simulink model "DT_enviroment_state_machine_llm_udp_simscape"  (R2026a)
settings: Solver=ode23t  StopTime=120.500  FixedStep=1e-3
InitFcn:
  | V_bias_cmd=0;
  | enable_cmd=0;
  | mode_cmd=0;
  | P_batt_cmd=0;
libraries: fl_lib x14, nesl_utility x12, batteryecm_lib x2, eeGeneralControl x2, slpidlib x2
(part 1 of 2)
settings Model: Creator=Peska  LastModifiedBy=thienan
settings DebuggingCC: SaveWithParameterizedLinksMsg=none
settings SimscapeCC: SimscapeLogType=none  SimscapeLogDataHistory=5000.0

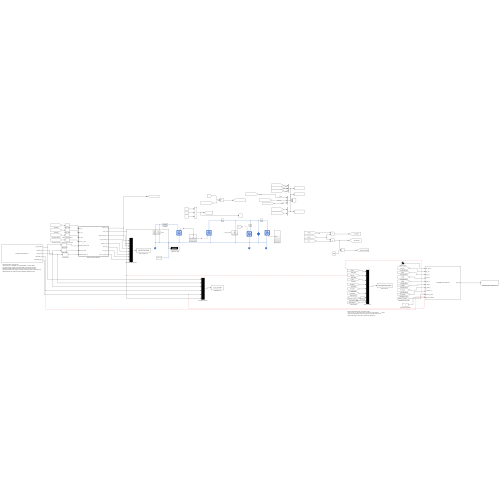
[thumbnail: Simulink's stored preview of the top-level diagram]
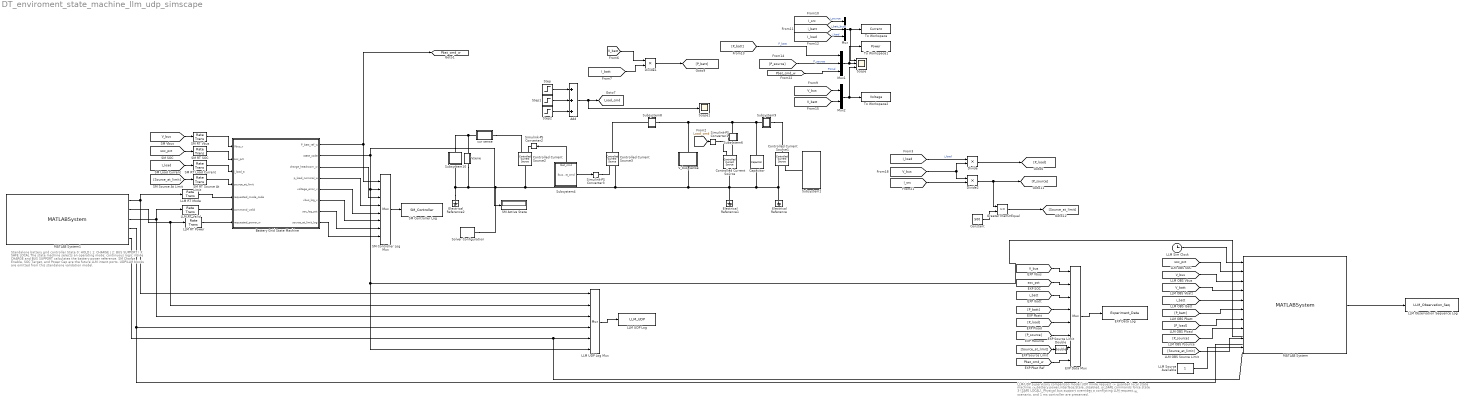
== system DT_enviroment_state_machine_llm_udp_simscape ==
  note: Standalone battery grid controller
      | State 0: HOLD | 1: CHARGE | 2: BUS SUPPORT | 3: SAFE LOCAL
      | The state machine selects an operating mode; continuous logic inside
      | CHARGE and BUS SUPPORT calculates the battery power reference.
      | SM Charge Enable, SOC Target, and Power Cap are the future LLM intent ports.
      | UDP/LLM blocks are omitted from this standalone validation model.
  note: Instrumented deterministic comparison model
      | This is a copy; DT_enviroment_state_machine.slx is unchanged.
      | The plant, state machine, scenario, and 1 ms controller are preserved.
  note: LLM/UDP supervisory comparison model
      | UDP mode request -> guarded local state machine -> battery power interface
      | Stale, disabled, or SAFE commands force state 3 (SAFE LOCAL).
      | Physical bus support overrides a conflicting LLM request.
  Add : Sum  Inputs=+++
  Battery Grid State Machine : MATLAB Function  TreatAsAtomicUnit=on
  Capacitor : fl_lib/Electrical/Electrical Elements/Capacitor  c=5e-3 F  r=1e-6 Ohm  g=0 1/Ohm  i_specify=off  i_priority=None  i=0 A  i_nominal_specify=off  i_nominal_value=1  i_nominal_unit=A  v_specify=off  v_priority=High  v=400 V  v_nominal_specify=off  v_nominal_value=1  v_nominal_unit=V  vc_specify=on  vc_priority=High  vc=400 V  vc_nominal_specify=off  vc_nominal_value=400  vc_nominal_unit=V
  Constant : Constant  Value=500
  Controlled Current Source{,1..3} (4 alike) : fl_lib/Electrical/Electrical Sources/Controlled Current Source
  Divide : Product  Inputs=**
  Divide1 : Product  Inputs=**
  Divide2 : Product  Inputs=**
  EXP Data Log : ToWorkspace  VariableName=Experiment_Data  SaveFormat=Structure With Time  SampleTime=-1
  EXP Data Mux : Mux  Inputs=8
  EXP Source Limit Double : DataTypeConversion  OutDataTypeStr=double  SaturateOnIntegerOverflow=off  RndMeth=Floor
  Electrical Reference : fl_lib/Electrical/Electrical Elements/Electrical Reference
  Electrical Reference1 : fl_lib/Electrical/Electrical Elements/Electrical Reference
  Electrical Reference2 : fl_lib/Electrical/Electrical Elements/Electrical Reference
  GreaterThanOrEqual : RelationalOperator  OutDataTypeStr=boolean  RndMeth=Simplest  InputSameDT=off
  LLM Observation Sequence Log : ToWorkspace  VariableName=LLM_Observation_Seq  SaveFormat=Structure With Time  SampleTime=-1
  LLM RT Mode : RateTransition  OutPortSampleTime=1e-3
  LLM RT Power : RateTransition  OutPortSampleTime=1e-3
  LLM RT Valid : RateTransition  OutPortSampleTime=1e-3
  LLM Sim Clock : Clock
  LLM Source Available : Constant
  LLM UDP Log : ToWorkspace  VariableName=LLM_UDP  SaveFormat=Structure With Time  SampleTime=-1
  LLM UDP Log Mux : Mux  Inputs=6
  MATLAB System : MATLABSystem  System=DTUdpObservationSender  RemoteHost=127.0.0.1  RemotePort=55001  SourceName=simulink  SampleDecimation=1  SourcePowerLimitW=NaN  MaxSafeChargeW=NaN
      mask Type: DTUdpObservationSender
  MATLAB System1 : MATLABSystem  System=DTUdpCommandReceiver  LocalPort=55000  DefaultPCommandW=0  DefaultEnable=on  DefaultModeCode=0  MaxCommandAgeS=10
      mask Type: DTUdpCommandReceiver
  Mux : Mux  Inputs=3
  Mux1 : Mux  Inputs=3
  Mux2 : Mux  Inputs=2
  SM Active State : Display
  SM Controller Log : ToWorkspace  VariableName=SM_Controller  SaveFormat=Structure With Time  SampleTime=-1
  SM Controller Log Mux : Mux  Inputs=8
  SM RT Load Current : RateTransition  OutPortSampleTime=1e-3
  SM RT SOC : RateTransition  OutPortSampleTime=1e-3
  SM RT Source At Limit : RateTransition  OutPortSampleTime=1e-3
  SM RT Vbus : RateTransition  OutPortSampleTime=1e-3
  Scope : Scope  NumInputPorts=3
      settings: TimeSpan=200  ActiveDisplayYMinimum=-1.87953  ActiveDisplayYMaximum=1.91579
  Scope1 : Scope
      settings: ActiveDisplayYMinimum=0.40625  ActiveDisplayYMaximum=1.34375
  Simulink-PS Converter1 : nesl_utility/Simulink-PS Converter  PhysicalDomain=network_engine_domain  SubClassName=ps_input  LeftPortType=input  RightPortType=output  PseudoPeriodic=off  Frequencies=[]  NoiseDistribution=none  NoiseParameters=[]  Unit=1  AffineConversion=off  FilteringAndDerivatives=provide  SimscapeFilterOrder=1  InputFilterTimeConstant=0.001  UdotUserProvided=0
  Simulink-PS Converter2 : nesl_utility/Simulink-PS Converter  PhysicalDomain=network_engine_domain  SubClassName=ps_input  LeftPortType=input  RightPortType=output  PseudoPeriodic=off  Frequencies=[]  NoiseDistribution=none  NoiseParameters=[]  Unit=1  AffineConversion=off  FilteringAndDerivatives=provide  SimscapeFilterOrder=1  InputFilterTimeConstant=0.001  UdotUserProvided=0
  Simulink-PS Converter3 : nesl_utility/Simulink-PS Converter  PhysicalDomain=network_engine_domain  SubClassName=ps_input  LeftPortType=input  RightPortType=output  PseudoPeriodic=off  Frequencies=[]  NoiseDistribution=none  NoiseParameters=[]  Unit=1  AffineConversion=off  FilteringAndDerivatives=provide  SimscapeFilterOrder=1  InputFilterTimeConstant=0.001  UdotUserProvided=0
  Solver Configuration : nesl_utility/Solver Configuration  PhysicalDomain=network_engine_domain  SubClassName=solver  LeftPortType=input  RightPortType=generic  Tones=[]  Harmonics=[]  SimulateNoise=off  Profile=off  UseLocalSampling=off  EnableSwitchedLinearOptims=on  FrequencyDomain=off  UseCCode=off  RelTol=0.001  AbsTol=0.001  MinStep=1e-09  ToWorkspace=off  RevertToSquareIcSolve=off  NumHomotopyIterations=100  PhasorMode=off  PhasorModeNumHarmonics=1  ConsistencySolver=NEWTON_XTOL_AFTER_FTOL  CanonicalOrdering=UNORDERED  OptimizeIntermediates=UNOPTIMIZED  IndexReductionMethod=DerivativeReplacement  DoDC=off  ResidualTolerance=1e-09  ConsistencyTolSource=GLOBAL  ConsistencyAbsTol=0.001  ConsistencyRelTol=0.001  ConsistencyTolFactor=0.001  UseLocalSolver=off  LocalSolverChoice=NE_BACKWARD_EULER_ADVANCER  ResolveIndetEquations=on  FunctionEvalNumThread=1  LocalSolverSampleTime=0.001  DoFixedCost=off  MaxNonlinIter=3  MaxModeIter=2  ComputeImpulses=off  ImpulseIterations=2  LinearAlgebra=auto  LinearAlgebraNumThread=0  EquationFormulation=NE_TIME_EF  DelaysMemoryBudget=1024  AutomaticFiltering=on  FilteringTimeConstant=0.001  PartitionStorageMethod=AS_NEEDED  PartitionMemoryBudget=1024  PartitionMethod=ROBUST  MultibodyUseLocalSolver=off  MultibodyLocalSolverChoice=ODE1  MultibodyLocalSolverSampleTime=0.001
  Step : Step  Time=50  InitialValue=0.5  FinalValue=1.25  SampleTime=0
  Step1 : Step  Time=100  FinalValue=0.25  SampleTime=0
  Step2 : Step  Time=160  FinalValue=-1  SampleTime=0
  Subsystem1 : Subsystem
  Subsystem10 : Subsystem
  Subsystem4 : Subsystem
      settings: PortSchema="{\"entries\":[{\"content\":{\"sides\":[{\"content\":{},\"type\":\"ConnectorPlacement.EquallySpacedRectSide\",\"uuid\":\"6a1a1ce4-53ed-4982-894a-a22a93ba5ab9\"},{\"content\":{\"connectorIds\":[\"Out1\"],\"side\":\"RIGHT\"},\"type\":\"ConnectorPlacement.EquallySpacedRectSide\",\"uuid\":\"d093341d-d8fd-41c9-a305-3247a499ae5f\"},{\"content\":{\"connectorIds\":[\"Out2\"],\"side\":\"TOP\"},\"type\":\"ConnectorPlacement.EquallySpacedRectSide\",\"uuid\":\"086192a8-14eb-4f6e-a910-e0970e09cefc\"}]},\"type\":\"ConnectorPlacement.EquallySpacedConnector\",\"uuid\":\"525000e1-7abd-43b8-b1b1-a1c81a980189\"}],\"packageUris\":[\"http://schema.mathworks.com/mf0/Connector/R2020b\"],\"version\":\"1.0\"}"
  Subsystem6 : Subsystem
  Subsystem8 : Subsystem
  Subsystem9 : Subsystem
  To Workspace : ToWorkspace  VariableName=Current  SampleTime=-1
      settings: Save2DSignal=2-D array (concatenate along first dimension)
  To Workspace1 : ToWorkspace  VariableName=Power  SampleTime=-1
      settings: Save2DSignal=2-D array (concatenate along first dimension)
  To Workspace2 : ToWorkspace  VariableName=Voltage  SampleTime=-1
      settings: Save2DSignal=2-D array (concatenate along first dimension)
  V_bus_sense : Subsystem
      settings: PortSchema="{\"entries\":[{\"content\":{\"sides\":[{\"content\":{},\"type\":\"ConnectorPlacement.EquallySpacedRectSide\",\"uuid\":\"8fde0f3a-65e7-4a5d-bf82-e35c7aed47e6\"},{\"content\":{\"side\":\"RIGHT\"},\"type\":\"ConnectorPlacement.EquallySpacedRectSide\",\"uuid\":\"008c88e1-cd0d-4683-93e1-f65f0bc6c32d\"},{\"content\":{\"connectorIds\":[\"LConn1\"],\"side\":\"TOP\"},\"type\":\"ConnectorPlacement.EquallySpacedRectSide\",\"uuid\":\"54cd5226-ad4a-4507-8beb-2e308d185250\"},{\"content\":{\"connectorIds\":[\"RConn1\"],\"side\":\"BOTTOM\"},\"type\":\"ConnectorPlacement.EquallySpacedRectSide\",\"uuid\":\"0d0454d8-66f2-48c0-bbc2-202193e06aa7\"}]},\"type\":\"ConnectorPlacement.EquallySpacedConnector\",\"uuid\":\"3936b8d3-7fc1-45c6-9850-1e68fec0f3da\"}],\"packageUris\":[\"http://schema.mathworks.com/mf0/Connector/R2020b\"],\"version\":\"1.0\"}"
  Vsene : Subsystem
      settings: PortSchema="{\"entries\":[{\"content\":{\"sides\":[{\"content\":{},\"type\":\"ConnectorPlacement.EquallySpacedRectSide\",\"uuid\":\"b9c82097-dbe0-4c7d-a854-e8918b3e4e62\"},{\"content\":{\"side\":\"RIGHT\"},\"type\":\"ConnectorPlacement.EquallySpacedRectSide\",\"uuid\":\"e6a2493d-d328-4064-a211-f9d94d1b4401\"},{\"content\":{\"connectorIds\":[\"LConn1\"],\"side\":\"TOP\"},\"type\":\"ConnectorPlacement.EquallySpacedRectSide\",\"uuid\":\"d04b113b-a585-4598-ab40-82f3ac9d078a\"},{\"content\":{\"connectorIds\":[\"RConn1\"],\"side\":\"BOTTOM\"},\"type\":\"ConnectorPlacement.EquallySpacedRectSide\",\"uuid\":\"e96f8fbf-f009-4596-a1dc-5ff08614d8bd\"}]},\"type\":\"ConnectorPlacement.EquallySpacedConnector\",\"uuid\":\"c6aac4e2-1941-41cc-b5dc-ae78ef227dce\"}],\"packageUris\":[\"http://schema.mathworks.com/mf0/Connector/R2020b\"],\"version\":\"1.0\"}"
  cur sense : Subsystem
  tag scope: Load_cmd=global, Pbat_cmd_w=global
  wires:
  [I_src] -> Mux/1  "i_source"
  [i_batt] -> Mux/2  "i_batt_buss"
  [I_load] -> Mux/3  "i_load"
  Mux/1 -> To Workspace/1, Scope/1
  [P_source] -> Mux1/2  "P_source"
  Mux1/1 -> To Workspace1/1, Scope/2
  [V_bus] -> Mux2/1
  [V_batt] -> Mux2/2
  Mux2/1 -> Scope/3, To Workspace2/1
  [I_load] -> Divide/1  "i_load"
  [V_bus] -> Divide2/1, Divide/2
  Divide/1 -> [P_load]
  [Pbat_cmd_w] -> Mux1/3  "Pcmd"
  [Load_cmd] -> Simulink-PS Converter1/1
  Subsystem4/1(Ibus_batt_cmd) -> Simulink-PS Converter3/1
  Subsystem4/2(Ibat_cmd) -> Simulink-PS Converter2/1
  [V_batt] -> Divide1/1
  [I_batt] -> Divide1/2
  Divide1/1 -> [P_batt]
  [I_src] -> Divide2/2
  Divide2/1 -> GreaterThanOrEqual/1, [P_source]
  GreaterThanOrEqual/1 -> [Source_at_limit]
  Constant/1 -> GreaterThanOrEqual/2
  Step1/1 -> Add/2
  Step/1 -> Add/1
  Add/1 -> Scope1/1, [Load_cmd]
  [P_batt] -> Mux1/1  "P_batt"
  [V_bus] -> SM RT Vbus/1
  SM RT Vbus/1 -> Battery Grid State Machine/1(Vbus_v)
  [soc_pct] -> SM RT SOC/1
  SM RT SOC/1 -> Battery Grid State Machine/2(soc_pct)
  [I_load] -> SM RT Load Current/1
  SM RT Load Current/1 -> Battery Grid State Machine/3(i_load_a)
  [Source_at_limit] -> SM RT Source At Limit/1
  SM RT Source At Limit/1 -> Battery Grid State Machine/4(source_at_limit)
  Battery Grid State Machine/1(P_batt_ref_w) -> SM Controller Log Mux/1, [Pbat_cmd_w]
  Battery Grid State Machine/2(state_code) -> SM Controller Log Mux/2, LLM UDP Log Mux/6, SM Active State/1
  Battery Grid State Machine/3(charge_headroom_w) -> SM Controller Log Mux/3
  Battery Grid State Machine/4(p_load_nominal_w) -> SM Controller Log Mux/4
  Battery Grid State Machine/5(voltage_error_v) -> SM Controller Log Mux/5
  Battery Grid State Machine/6(vbus_log_v) -> SM Controller Log Mux/6
  Battery Grid State Machine/7(soc_log_pct) -> SM Controller Log Mux/7
  Battery Grid State Machine/8(source_at_limit_log) -> SM Controller Log Mux/8
  SM Controller Log Mux/1 -> SM Controller Log/1
  [V_bus] -> EXP Data Mux/1
  [soc_pct] -> EXP Data Mux/2
  [i_batt] -> EXP Data Mux/3
  [P_batt] -> EXP Data Mux/4
  [P_load] -> EXP Data Mux/5
  [P_source] -> EXP Data Mux/6
  [Source_at_limit] -> EXP Source Limit Double/1
  EXP Source Limit Double/1 -> EXP Data Mux/7
  [Pbat_cmd_w] -> EXP Data Mux/8
  EXP Data Mux/1 -> EXP Data Log/1
  MATLAB System1/1 -> LLM RT Mode/1, LLM UDP Log Mux/1
  LLM RT Mode/1 -> Battery Grid State Machine/5(requested_mode_code)
  MATLAB System1/3 -> LLM UDP Log Mux/3, LLM RT Valid/1
  LLM RT Valid/1 -> Battery Grid State Machine/6(command_valid)
  MATLAB System1/2 -> LLM RT Power/1, LLM UDP Log Mux/2
  LLM RT Power/1 -> Battery Grid State Machine/7(requested_power_w)
  MATLAB System1/4 -> LLM UDP Log Mux/4
  MATLAB System1/5 -> LLM UDP Log Mux/5
  LLM UDP Log Mux/1 -> LLM UDP Log/1
  LLM Sim Clock/1 -> MATLAB System/1
  [soc_pct] -> MATLAB System/2
  [V_bus] -> MATLAB System/3
  [V_batt] -> MATLAB System/4
  [i_batt] -> MATLAB System/5
  [P_batt] -> MATLAB System/6
  [P_load] -> MATLAB System/7
  [P_source] -> MATLAB System/8
  [Source_at_limit] -> MATLAB System/9
  LLM Source Available/1 -> MATLAB System/10
  MATLAB System/1 -> LLM Observation Sequence Log/1
  Step2/1 -> Add/3
  connections:
  Subsystem8/LConn1 -- Capacitor/LConn1 -- Subsystem9/LConn1 -- Subsystem6/LConn1 -- V_bus_sense/LConn1
  Electrical Reference2/LConn1 -- Subsystem10/RConn1 -- Vsene/RConn1 -- Controlled Current Source1/RConn2 -- Electrical Reference/LConn1 -- Capacitor/RConn1 -- Electrical Reference1/LConn1 -- Controlled Current Source/LConn1 -- V_bus_sense/RConn1 -- Controlled Current Source3/RConn2 -- Controlled Current Source2/LConn1 -- Solver Configuration/RConn1
  Subsystem10/LConn1 -- cur sense/LConn1 -- Vsene/LConn1
  Simulink-PS Converter1/RConn1 -- Controlled Current Source/RConn1
  Controlled Current Source/RConn2 -- Subsystem6/RConn1
  Simulink-PS Converter3/RConn1 -- Controlled Current Source3/RConn1
  Controlled Current Source2/RConn1 -- Simulink-PS Converter2/RConn1
  Subsystem9/RConn1 -- Controlled Current Source1/LConn1
  Subsystem8/RConn1 -- Controlled Current Source3/LConn1
  cur sense/RConn1 -- Controlled Current Source2/RConn2
  Controlled Current Source1/RConn1 -- Subsystem1/RConn1

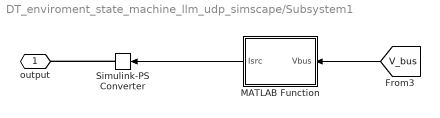
== system DT_enviroment_state_machine_llm_udp_simscape/Subsystem1 ==
  MATLAB Function : MATLAB Function  TreatAsAtomicUnit=on
  Simulink-PS Converter : nesl_utility/Simulink-PS Converter  PhysicalDomain=network_engine_domain  SubClassName=ps_input  LeftPortType=input  RightPortType=output  PseudoPeriodic=off  Frequencies=[]  NoiseDistribution=none  NoiseParameters=[]  Unit=1  AffineConversion=off  FilteringAndDerivatives=provide  SimscapeFilterOrder=1  InputFilterTimeConstant=0.001  UdotUserProvided=0
  output : PMIOPort  Side=Right
  wires:
  [V_bus] -> MATLAB Function/1(Vbus)
  MATLAB Function/1(Isrc) -> Simulink-PS Converter/1
  connections:
  Simulink-PS Converter/RConn1 -- output/RConn1

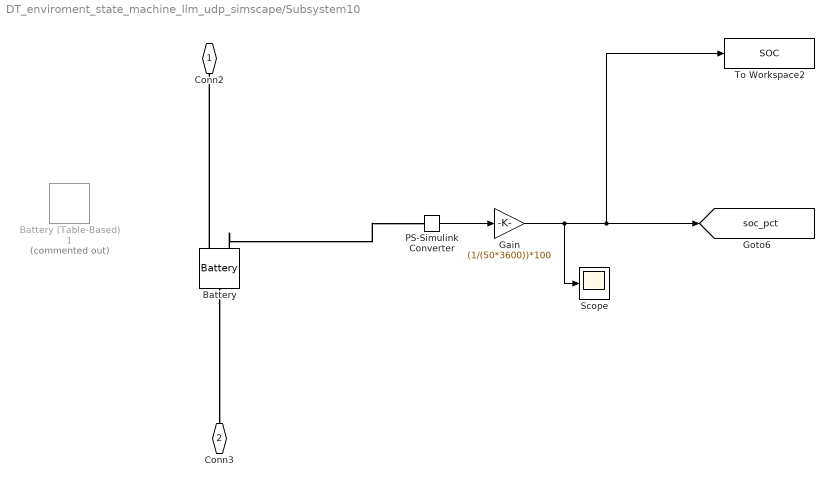
== system DT_enviroment_state_machine_llm_udp_simscape/Subsystem10 ==
  Battery : batteryecm_lib/Battery  Vnom=300 V  prm_dir=simscape.enum.battery.prm_dir.disabled  R1_dis=2 Ohm  R1_ch=2 Ohm  R1=2 Ohm  prm_AH=simscape.enum.battery.prm_AH.finite  AH=50 A*hr  V1=295 V  AH1=25 A*hr  prm_R2=simscape.enum.battery.prm_R2.disabled  R2=2000 Ohm  Tmeas=298.15 K  charge_measurement_port=simscape.enum.battery.enable.yes  prm_dyn=simscape.enum.battery.prm_dyn.off  Rp1=0.005 Ohm  tau1=30 s  Rp2=0.005 Ohm  tau2=30 s  Rp3=0.005 Ohm  tau3=30 s  Rp4=0.005 Ohm  tau4=30 s  Rp5=0.005 Ohm  tau5=30 s  prm_fade=simscape.enum.battery.prm_fade.disabled  N_fade=100  AH_fade=45 A*hr  R1_fade=2.02 Ohm  R1_ch_fade=2.02 Ohm  V1_fade=10.35 V  prm_age=simscape.enum.battery.prm_age.disabled  prm_age_OCV=simscape.enum.battery.prm_age_OCV.OCV  OCV_age=0.9  SOC_age=60  Tmeas_age=298.15 K  delta_time_age_vec=[0] d  temperature_age_vec=[273] K  OCV_scaling_age=2.2134e6  OCV_offset_age=1.632e6  temp_exp_age=0.515833569 V  t_exp_age=0.75  Vnom_T2=12 V  R1_T2=2.2 Ohm  R1_T2_dis=2.2 Ohm  R1_T2_ch=2.2 Ohm  V1_T2=11.4 V  R2_T2=2200 Ohm  Rp1_T2=0.005 Ohm  tau1_T2=30 s  Rp2_T2=0.005 Ohm  tau2_T2=30 s  Rp3_T2=0.005 Ohm  tau3_T2=30 s  Rp4_T2=0.005 Ohm  tau4_T2=30 s  Rp5_T2=0.005 Ohm  tau5_T2=30 s  Tmeas2=273.15 K  thermal_port=simscape.enum.thermaleffects.omit  thermal_mass=30000 J/K  i_specify=off  i_priority=None  i=0 A  i_nominal_specify=off  i_nominal_value=1  i_nominal_unit=A  v_specify=off  v_priority=None  v=0 V  v_nominal_specify=off  v_nominal_value=1  v_nominal_unit=V  charge_specify=on  charge_priority=High  charge=50*0.15 A*hr  charge_nominal_specify=off  charge_nominal_value=1  charge_nominal_unit=A*hr  num_cycles_specify=off  num_cycles_priority=High  num_cycles=0  num_cycles_nominal_specify=off  num_cycles_nominal_value=1  num_cycles_nominal_unit=1  temperature_specify=off  temperature_priority=High  temperature=298.15 K  temperature_nominal_specify=off  temperature_nominal_value=1  temperature_nominal_unit=K
  Battery (Table-Based)1 : batteryecm_lib/Battery (Table-Based)  Commented=on  PartSpecification="{\"DatasetId\":\"Valence|U27_36XP|simscape.battery.batteryTableBased\",\"DisplayName\":\"Valence:U27_36XP\"}"  SOC_vec=[0 0.01 0.02 0.03 0.04 0.05 0.06 0.07 0.08 0.09 0.1 0.11 0.12 0.13 0.14 0.15 0.16 0.17 0.18 0.19 0.2 0.21 0.22 0.23 0.24 0.25 0.26 0.27 0.28 0.29 0.3 0.31 0.32 0.33 0.34 0.35 0.36 0.37 0.38 0.39 0.4 0.41 0.42 0.43 0.44 0.45 0.46 0.47 0.48 0.49 0.5 0.51 0.52 0.53 0.54 0.55 0.56 0.57 0.58 0.59 0.6 0.61 0.62 0.63 0.64 0.65 0.66 0.67 0.68 0.69 0.7 0.71 0.72 0.73 0.74 0.75 0.76 0.77 0.78 0.79 0.8 0.81 0.82 0.83 0.84 0.85 0.86 0.87 0.88 0.89 0.9 0.91 0.92 0.93 0.94 0.95 0.96 0.97 0.98 0.99 1] % Datasheet derived  T_dependence=simscape.enum.tablebattery.temperature_dependence.yes  prm_dir=simscape.enum.tablebattery.prm_dir.noCurrentDirectionality  T_vec=[-10 0 10 20 23 30 40 50] % Datasheet derived degC  V0_mat=[35.84591 35.84591 35.84591 35.84591 35.84591 35.84591 35.84591 35.84591;36.10202 36.10202 36.10202 36.10202 36.10202 36.10202 36.10202 36.10202;36.35814 36.35814 36.35814 36.35814 36.35814 36.35814 36.35814 36.35814;36.61425 36.61425 36.61425 36.61425 36.61425 36.61425 36.61425 36.61425;36.87037 36.87037 36.87037 36.87037 36.87037 36.87037 36.87037 36.87037;37.12649 37.12649 37.12649 37.12649 37.12649 37.12649 37.12649 37.12649;37.3826 37.3826 37.3826 37.3826 37.3826 37.3826 37.3826 37.3826;37.63872 37.63872 37.63872 37.63872 37.63872 37.63872 37.63872 37.63872;37.89483 37.89483 37.89483 37.89483 37.89483 37.89483 37.89483 37.89483;38.09951 38.09951 38.09951 38.09951 38.09951 38.09951 38.09951 38.09951;38.20904 38.20904 38.20904 38.20904 38.20904 38.20904 38.20904 38.20904;38.28916 38.28916 38.28916 38.28916 38.28916 38.28916 38.28916 38.28916;38.37306 38.37306 38.37306 38.37306 38.37306 38.37306 38.37306 38.37306;38.42308 38.42308 38.42308 38.42308 38.42308 38.42308 38.42308 38.42308;38.45482 38.45482 38.45482 38.45482 38.45482 38.45482 38.45482 38.45482;38.47744 38.47744 38.47744 38.47744 38.47744 38.47744 38.47744 38.47744;38.49779 38.49779 38.49779 38.49779 38.49779 38.49779 38.49779 38.49779;38.54815 38.54815 38.54815 38.54815 38.54815 38.54815 38.54815 38.54815;38.5883 38.5883 38.5883 38.5883 38.5883 38.5883 38.5883 38.5883;38.63829 38.63829 38.63829 38.63829 38.63829 38.63829 38.63829 38.63829;38.68732 38.68732 38.68732 38.68732 38.68732 38.68732 38.68732 38.68732;38.72975 38.72975 38.72975 38.72975 38.72975 38.72975 38.72975 38.72975;38.77111 38.77111 38.77111 38.77111 38.77111 38.77111 38.77111 38.77111;38.80795 38.80795 38.80795 38.80795 38.80795 38.80795 38.80795 38.80795;38.83724 38.83724 38.83724 38.83724 38.83724 38.83724 38.83724 38.83724;38.8617 38.8617 38.8617 38.8617 38.8617 38.8617 38.8617 38.8617;38.89023 38.89023 38.89023 38.89023 38.89023 38.89023 38.89023 38.89023;38.9273 38.9273 38.9273 38.9273 38.9273 38.9273 38.9273 38.9273;38.96054 38.96054 38.96054 38.96054 38.96054 38.96054 38.96054 38.96054;38.98786 38.98786 38.98786 38.98786 38.98786 38.98786 38.98786 38.98786;39.01519 39.01519 39.01519 39.01519 39.01519 39.01519 39.01519 39.01519;39.03864 39.03864 39.03864 39.03864 39.03864 39.03864 39.03864 39.03864;39.06385 39.06385 39.06385 39.06385 39.06385 39.06385 39.06385 39.06385;39.08223 39.08223 39.08223 39.08223 39.08223 39.08223 39.08223 39.08223;39.1006 39.1006 39.1006 39.1006 39.1006 39.1006 39.1006 39.1006;39.11898 39.11898 39.11898 39.11898 39.11898 39.11898 39.11898 39.11898;39.13735 39.13735 39.13735 39.13735 39.13735 39.13735 39.13735 39.13735;39.15508 39.15508 39.15508 39.15508 39.15508 39.15508 39.15508 39.15508;39.16412 39.16412 39.16412 39.16412 39.16412 39.16412 39.16412 39.16412;39.17437 39.17437 39.17437 39.17437 39.17437 39.17437 39.17437 39.17437;39.18528 39.18528 39.18528 39.18528 39.18528 39.18528 39.18528 39.18528;39.19619 39.19619 39.19619 39.19619 39.19619 39.19619 39.19619 39.19619;39.20709 39.20709 39.20709 39.20709 39.20709 39.20709 39.20709 39.20709;39.21696 39.21696 39.21696 39.21696 39.21696 39.21696 39.21696 39.21696;39.22232 39.22232 39.22232 39.22232 39.22232 39.22232 39.22232 39.22232;39.22753 39.22753 39.22753 39.22753 39.22753 39.22753 39.22753 39.22753;39.23277 39.23277 39.23277 39.23277 39.23277 39.23277 39.23277 39.23277;39.23672 39.23672 39.23672 39.23672 39.23672 39.23672 39.23672 39.23672;39.23942 39.23942 39.23942 39.23942 39.23942 39.23942 39.23942 39.23942;39.24211 39.24211 39.24211 39.24211 39.24211 39.24211 39.24211 39.24211;39.24481 39.24481 39.24481 39.24481 39.24481 39.24481 39.24481 39.24481;39.24786 39.24786 39.24786 39.24786 39.24786 39.24786 39.24786 39.24786;39.25094 39.25094 39.25094 39.25094 39.25094 39.25094 39.25094 39.25094;39.2539 39.2539 39.2539 39.2539 39.2539 39.2539 39.2539 39.2539;39.25686 39.25686 39.25686 39.25686 39.25686 39.25686 39.25686 39.25686;39.26099 39.26099 39.26099 39.26099 39.26099 39.26099 39.26099 39.26099;39.26708 ...(+3199 chars)] % Datasheet derived V  V0_vec=[35.84591 36.10202 36.35814 36.61425 36.87037 37.12649 37.3826 37.63872 37.89483 38.09951 38.20904 38.28916 38.37306 38.42308 38.45482 38.47744 38.49779 38.54815 38.5883 38.63829 38.68732 38.72975 38.77111 38.80795 38.83724 38.8617 38.89023 38.9273 38.96054 38.98786 39.01519 39.03864 39.06385 39.08223 39.1006 39.11898 39.13735 39.15508 39.16412 39.17437 39.18528 39.19619 39.20709 39.21696 39.22232 39.22753 39.23277 39.23672 39.23942 39.24211 39.24481 39.24786 39.25094 39.2539 39.25686 39.26099 39.26708 39.27551 39.28394 39.29233 39.30067 39.31557 39.33487 39.35402 39.37113 39.38825 39.40815 39.43406 39.46187 39.48968 39.51913 39.55031 39.5817 39.60619 39.62271 39.63907 39.65521 39.67134 39.68137 39.69071 39.70005 39.7052 39.70868 39.70916 39.70862 39.70807 39.70752 39.71037 39.72142 39.72908 39.73651 39.73911 39.73577 39.72919 39.73278 39.7392 39.74638 39.75462 39.8136 40.01141 40.30627] % Datasheet derived V  V_range=[27 Inf] % Datasheet derived V  R0_mat=[0.9112 0.73319 0.55116 0.3909 0.47635 0.31145 0.24894 0.23351;0.9112 0.79214 0.50936 0.32708 0.41138 0.21289 0.15029 0.11642;0.9112 0.75838 0.46755 0.26325 0.35007 0.14203 0.09214 0.07324;0.9112 0.72463 0.42575 0.19942 0.29417 0.09634 0.05758 0.04021;0.9112 0.69087 0.38395 0.15149 0.24882 0.06764 0.03364 0.02182;0.9112 0.65711 0.34215 0.11725 0.2142 0.04885 0.01957 0.00983;0.9112 0.62335 0.30035 0.09581 0.18886 0.03484 0.01134 0.00372;0.88245 0.58959 0.25855 0.08105 0.17031 0.02886 0.01013 0.00445;0.85369 0.55583 0.22327 0.07125 0.1569 0.02915 0.01483 0.00976;0.82493 0.52207 0.19506 0.06386 0.14398 0.03152 0.0196 0.01392;0.79618 0.48831 0.16793 0.05824 0.13028 0.031 0.02172 0.01735;0.76742 0.45455 0.14437 0.05231 0.11716 0.03152 0.02306 0.0196;0.73866 0.42079 0.12447 0.04884 0.10632 0.03219 0.02454 0.02192;0.70991 0.38703 0.1096 0.04638 0.09512 0.03151 0.02458 0.0216;0.68115 0.35327 0.09525 0.04318 0.08414 0.02987 0.02387 0.02054;0.65239 0.31952 0.08121 0.03996 0.07347 0.02787 0.02226 0.01912;0.62364 0.27915 0.07388 0.03692 0.06467 0.02578 0.02045 0.01757;0.59488 0.24506 0.06774 0.03508 0.05964 0.02492 0.01984 0.01722;0.56612 0.21466 0.06284 0.03384 0.05477 0.02422 0.01882 0.01646;0.53737 0.18917 0.06009 0.03346 0.05154 0.02391 0.0187 0.0161;0.50861 0.16681 0.05729 0.03301 0.04841 0.02357 0.0188 0.0157;0.47986 0.14646 0.05423 0.03228 0.04625 0.02296 0.01864 0.01586;0.4511 0.13143 0.05231 0.0315 0.04448 0.02305 0.01844 0.01609;0.42234 0.11995 0.05123 0.03055 0.04297 0.02298 0.01851 0.01613;0.39359 0.10903 0.04985 0.03032 0.04112 0.02261 0.01828 0.01587;0.36483 0.09944 0.04828 0.02989 0.03908 0.02204 0.01786 0.01541;0.33607 0.09353 0.04687 0.02963 0.0378 0.02164 0.01762 0.01512;0.30291 0.08834 0.04648 0.02972 0.03771 0.02158 0.01779 0.01527;0.27067 0.08411 0.04619 0.02964 0.03746 0.0219 0.0178 0.01525;0.24264 0.08054 0.04566 0.02987 0.03699 0.02206 0.01758 0.015;0.21621 0.07803 0.04513 0.03012 0.03652 0.02222 0.01736 0.01476;0.19063 0.07544 0.04456 0.03022 0.03598 0.02223 0.01698 0.01435;0.17492 0.07417 0.04451 0.03039 0.03587 0.0223 0.01675 0.01402;0.15924 0.07263 0.04418 0.03029 0.03552 0.0221 0.01669 0.01376;0.14506 0.07109 0.04385 0.03019 0.03517 0.0219 0.01663 0.01361;0.13357 0.06955 0.04352 0.03009 0.03481 0.0217 0.01658 0.01346;0.12461 0.0686 0.04319 0.02998 0.03446 0.0215 0.01652 0.01331;0.11872 0.06771 0.04286 0.02995 0.03417 0.02128 0.01643 0.01313;0.11354 0.06648 0.04251 0.02967 0.03358 0.02084 0.016 0.01261;0.10849 0.0653 0.0422 0.02943 0.03336 0.02078 0.01562 0.01213;0.10559 0.06415 0.04193 0.02923 0.03321 0.02075 0.01526 0.01187;0.10269 0.06364 0.04165 0.02902 0.03305 0.02071 0.01515 0.01197;0.09978 0.06339 0.04137 0.02881 0.0329 0.02068 0.01521 0.01208;0.09733 0.06309 0.04105 0.02856 0.0327 0.0206 0.01523 0.01214;0.09518 0.06261 0.0406 0.02813 0.03227 0.02035 0.01507 0.01203;0.09303 0.06213 0.04031 0.0277 0.03186 0.02009 0.01491 0.01191;0.0912 0.06165 0.04003 0.02736 0.03148 0.01983 0.01474 0.01179;0.08999 0.06112 0.0397 0.02706 0.03105 0.01963 0.01452 0.01161;0.08874 0.06053 0.03932 0.02671 0.03058 0.0194 0.01426 0.01139;0.08749 0.05993 0.03893 0.02636 0.03011 0.01916 0.01399 0.01119;0.08652 0.05934 0.03855 0.02601 0.02964 0.01893 0.01372 0.01104;0.08605 0.05876 0.03818 0.02568 0.02918 0.01872 0.01346 0.01091;0.08557 0.05819 0.03788 0.02534 0.02875 0.0185 0.0132 0.01078;0.0851 0.0576 0.03759 0.025 0.02834 0.01828 0.01294 0.01065;0.08479 0.05702 0.0373 0.02466 0.02792 0.01806 0.01268 0.01051;0.08459 0.05663 0.03706 0.0244 0.02762 0.01789 0.01247 0.01042;0.08446 0.0566 0.0369 0.02423 0.02745 0.01779 0.01233 0.01038;0.08442 0.05667 0.03684 0.02414 0.02737 0.01779 0.01229 0.01018;0.08439 0.05674 0.03677 0.02406 0.02729 0.01777 0.01225 0.00997;0.08436 0.05681 0.0367 0.02397 0.02722 0.01767 0.01221 0.00977;0.08463 0.05687 0.03669 0.02389 0.02715 0.01757 0.01218 0.00956;0.08516 0.0572 0.03698 0.02406 0.0274 0.01773 0.0124 0.00962;0.08586 0.0577 0.03744 0.02442 0.02786 0.01806 0.0128 0.00985;0.08657 0.05819 0.0379 ...(+2382 chars)] % Datasheet derived Ohm  R0_vec=[0.47635 0.41138 0.35007 0.29417 0.24882 0.2142 0.18886 0.17031 0.1569 0.14398 0.13028 0.11716 0.10632 0.09512 0.08414 0.07347 0.06467 0.05964 0.05477 0.05154 0.04841 0.04625 0.04448 0.04297 0.04112 0.03908 0.0378 0.03771 0.03746 0.03699 0.03652 0.03598 0.03587 0.03552 0.03517 0.03481 0.03446 0.03417 0.03358 0.03336 0.03321 0.03305 0.0329 0.0327 0.03227 0.03186 0.03148 0.03105 0.03058 0.03011 0.02964 0.02918 0.02875 0.02834 0.02792 0.02762 0.02745 0.02737 0.02729 0.02722 0.02715 0.0274 0.02786 0.0283 0.02854 0.02877 0.02906 0.02956 0.03013 0.0307 0.03135 0.03204 0.03271 0.03308 0.03307 0.03314 0.03323 0.03332 0.03312 0.03288 0.03264 0.03224 0.03172 0.03113 0.03057 0.03001 0.02945 0.02905 0.02924 0.0293 0.02938 0.02923 0.02879 0.02803 0.02792 0.02793 0.02786 0.02652 0.02587 0.02701 0.00941] % Datasheet derived Ohm  R0_dis_mat=[.0117, .0085, .009; .011, .0085, .009; .0114, .0087, .0092; .0107, .0082, .0088; .0107, .0083, .0091; .0113, .0085, .0089; .0116, .0085, .0089] % Parameter not set Ohm  R0_dis_vec=[.0085, .0085, .0087, .0082, .0083, .0085, .0085] % Parameter not set Ohm  R0_ch_mat=[.0117, .0085, .009; .011, .0085, .009; .0114, .0087, .0092; .0107, .0082, .0088; .0107, .0083, .0091; .0113, .0085, .0089; .0116, .0085, .0089] % Parameter not set Ohm  R0_ch_vec=[.0085, .0085, .0087, .0082, .0083, .0085, .0085] % Parameter not set Ohm  AH=50.41 % Datasheet derived hr*A  prm_leak=simscape.enum.tablebattery.prm_leak.disabled  Rleak_vec=[8000, 7000, 6000] % Parameter not set Ohm  Rleak=7e3 % Parameter not set Ohm  extrapolation_option=simscape.enum.extrapolation.nearest  SOC_port=simscape.enum.tablebattery.enable.yes  prm_dyn=simscape.enum.tablebattery.prm_dyn.off  R1_mat=[.0109, .0029, .0013; .0069, .0024, .0012; .0047, .0026, .0013; .0034, .0016, .001; .0033, .0023, .0014; .0033, .0018, .0011; .0028, .0017, .0011] % Parameter not set Ohm  R1_vec=[.0029, .0024, .0026, .0016, .0023, .0018, .0017] % Parameter not set Ohm  tau1_mat=[20, 36, 39; 31, 45, 39; 109, 105, 61; 36, 29, 26; 59, 77, 67; 40, 33, 29; 25, 39, 33] % Parameter not set s  tau1_vec=[36, 45, 105, 29, 77, 33, 39] % Parameter not set s  R2_mat=[.0109, .0029, .0013; .0069, .0024, .0012; .0047, .0026, .0013; .0034, .0016, .001; .0033, .0023, .0014; .0033, .0018, .0011; .0028, .0017, .0011] % Parameter not set Ohm  R2_vec=[.0029, .0024, .0026, .0016, .0023, .0018, .0017] % Parameter not set Ohm  tau2_mat=[20, 36, 39; 31, 45, 39; 109, 105, 61; 36, 29, 26; 59, 77, 67; 40, 33, 29; 25, 39, 33] % Parameter not set s  tau2_vec=[36, 45, 105, 29, 77, 33, 39] % Parameter not set s  R3_mat=[.0109, .0029, .0013; .0069, .0024, .0012; .0047, .0026, .0013; .0034, .0016, .001; .0033, .0023, .0014; .0033, .0018, .0011; .0028, .0017, .0011] % Parameter not set Ohm  R3_vec=[.0029, .0024, .0026, .0016, .0023, .0018, .0017] % Parameter not set Ohm  tau3_mat=[20, 36, 39; 31, 45, 39; 109, 105, 61; 36, 29, 26; 59, 77, 67; 40, 33, 29; 25, 39, 33] % Parameter not set s  tau3_vec=[36, 45, 105, 29, 77, 33, 39] % Parameter not set s  R4_mat=[.0109, .0029, .0013; .0069, .0024, .0012; .0047, .0026, .0013; .0034, .0016, .001; .0033, .0023, .0014; .0033, .0018, .0011; .0028, .0017, .0011] % Parameter not set Ohm  R4_vec=[.0029, .0024, .0026, .0016, .0023, .0018, .0017] % Parameter not set Ohm  tau4_mat=[20, 36, 39; 31, 45, 39; 109, 105, 61; 36, 29, 26; 59, 77, 67; 40, 33, 29; 25, 39, 33] % Parameter not set s  tau4_vec=[36, 45, 105, 29, 77, 33, 39] % Parameter not set s  R5_mat=[.0109, .0029, .0013; .0069, .0024, .0012; .0047, .0026, .0013; .0034, .0016, .001; .0033, .0023, .0014; .0033, .0018, .0011; .0028, .0017, .0011] % Parameter not set Ohm  R5_vec=[.0029, .0024, .0026, .0016, .0023, .0018, .0017] % Parameter not set Ohm  tau5_mat=[20, 36, 39; 31, 45, 39; 109, 105, 61; 36, 29, 26; 59, 77, 67; 40, 33, 29; 25, 39, 33] % Parameter not set s  tau5_vec=[36, 45, 105, 29, 77, 33, 39] % Parameter not set s  prm_fade=simscape.enum.tablebattery.prm_fade.tableN  N0=100 % Parameter not set  dV0=0 % Parameter not set  dR0=0 % Parameter not set  dAH=0 % Parameter not set  dRleak=0 % Parameter not set  dR1=0 % Parameter not set  dR2=0 % Parameter not set  dR3=0 % Parameter not set  dR4=0 % Parameter not set  dR5=0 % Parameter not set  N0vec=[0 49 97 145 193 241 289 337 385 433 481 529 577 625 673 721 769 817 865 913 961 1009 1057 1105 1153 1201 1249 1297 1345 1393 1441 1489 1537 1585 1633 1681 1729 1777 1825 1873 1921 1969 2017 2065 2113 2161 2209 2257 2305 2353 2401 2449 2497 2545 2593 2641 2689 2737 2785 2833 2881 2929 2977 3025 3073 3121 3169 3217 3265 3313 3361 3409 3457 3505 3553 3601 3649 3697 3745 3793 3841 3889 3937 3985 4033 4081 4129 4177 4225 4273 4321 4369 4417 4465 4513 4561 4609 4657 4705 4753] % Datasheet derived  Tfadevec=[298.15, 323.15] % Parameter not set K  dV0vec=[0 -0.3454 -0.6908 -0.9359 -1.1676 -1.2672 -1.3271 -1.3712 -1.3796 -1.388 -1.3952 -1.402 -1.4086 -1.4146 -1.4207 -1.4251 -1.4284 -1.4315 -1.4266 -1.421 -1.4155 -1.4126 -1.4098 -1.4073 -1.4101 -1.4131 -1.4208 -1.4293 -1.4381 -1.447 -1.458 -1.4708 -1.4792 -1.4819 -1.4846 -1.4851 -1.4846 -1.4841 -1.4836 -1.483 -1.4824 -1.4819 -1.4816 -1.4821 -1.4826 -1.4864 -1.4903 -1.4956 -1.5014 -1.5097 -1.5201 -1.5313 -1.5437 -1.5564 -1.5697 -1.5877 -1.609 -1.6303 -1.6517 -1.6733 -1.6925 -1.7109 -1.7294 -1.7531 -1.7804 -1.8107 -1.8457 -1.8808 -1.9156 -1.9505 -1.9835 -2.0164 -2.048 -2.0852 -2.1232 -2.1613 -2.1969 -2.2314 -2.2586 -2.2847 -2.3081 -2.3315 -2.3541 -2.3775 -2.4018 -2.4263 -2.4508 -2.4714 -2.4903 -2.5029 -2.5135 -2.5281 -2.5444 -2.5606 -2.5769 -2.589 -2.5984 -2.6056 -2.6113 -2.617] % Datasheet derived  dR0vec=[0 0 0 0 0 0 0 0 0 0 0 0 0 0 0 0 0 0 0 0 0 0 0 0 0 0 0 0 0 0 0 0 0 0 0 0 0 0 0 0 0 0 0 0 0 0 0 0 0 0 0 0 0 0 0 0 0 0 0 0 0 0 0 0 0 0 0 0 0 0 0 0 0 0 0 0 0 0 0 0 0 0 0 0 0 0 0 0 0 0 0 0 0 0 0 0 0 0 0 0] % Parameter assumed  dAHvec=[0 -0.472 -0.944 -1.416 -1.889 -2.306 -2.716 -3.125 -3.535 -3.944 -4.342 -4.723 -5.104 -5.485 -5.867 -6.248 -6.629 -6.972 -7.314 -7.656 -7.997 -8.339 -8.681 -9.022 -9.457 -9.923 -10.389 -10.855 -11.321 -11.787 -12.254 -12.72 -13.106 -13.491 -13.876 -14.262 -14.647 -15.032 -15.417 -15.837 -16.264 -16.69 -17.116 -17.542 -17.987 -18.438 -18.889 -19.341 -19.792 -20.243 -20.694 -21.177 -21.71 -22.243 -22.776 -23.309 -23.842 -24.376 -24.909 -25.442 -25.915 -26.366 -26.816 -27.266 -27.717 -28.167 -28.617 -29.068 -29.518 -29.968 -30.419 -30.869 -31.319 -31.858 -32.41 -32.961 -33.512 -34.063 -34.615 -35.166 -35.717 -36.269 -36.802 -37.314 -37.826 -38.339 -38.851 -39.363 -39.875 -40.388 -40.9 -41.603 -42.38 -43.158 -43.935 -44.712 -45.49 -46.267 -47.044 -47.822] % Datasheet derived  dRleakvec=[0, 0, 0, 0] % Parameter not set  dR1vec=[0, 0, 0, 0] % Parameter not set  dR2vec=[0, 0, 0, 0] % Parameter not set  dR3vec=[0, 0, 0, 0] % Parameter not set  dR4vec=[0, 0, 0, 0] % Parameter not set  dR5vec=[0, 0, 0, 0] % Parameter not set  dV0mat=[0, 0; 0, 0; 0, 0; 0, 0] % Parameter not set  dR0mat=[0, 0; 0, 0; 0, 0; 0, 0] % Parameter not set  dAHmat=[0, 0; 0, 0; 0, 0; 0, 0] % Parameter not set  dRleakmat=[0, 0; 0, 0; 0, 0; 0, 0] % Parameter not set  dR1mat=[0, 0; 0, 0; 0, 0; 0, 0] % Parameter not set  dR2mat=[0, 0; 0, 0; 0, 0; 0, 0] % Parameter not set  dR3mat=[0, 0; 0, 0; 0, 0; 0, 0] % Parameter not set  dR4mat=[0, 0; 0, 0; 0, 0; 0, 0] % Parameter not set  dR5mat=[0, 0; 0, 0; 0, 0; 0, 0] % Parameter not set  prm_age_modeling=simscape.enum.tablebattery.prm_age_modeling.equation  storage_dt_age_vec=[0] % Parameter not set d  storage_T_age_vec=[273] % Parameter not set K  prm_age_OCV=simscape.enum.tablebattery.prm_age_OCV.OCV  OCV_age=0.9 % Parameter not set  SOC_age=0.6 % Parameter not set  prm_age_resistance=simscape.enum.tablebattery.prm_age.disabled  OCV_scaling_age_resistance=2.2134e6 % Parameter not set  OCV_offset_age_resistance=1.632e6 % Parameter not set  temp_exp_age_resistance=0.515833569 % Parameter not set V  t_exp_age_resistance=0.75 % Parameter not set  T_age_vec_resistance=[273.15, 298.15, 323.15] % Parameter not set K  dt_age_vec_resistance=[0, 90, 180, 270] % Parameter not set d  dR0_age_vec=[0, 0, 0] % Parameter not set  t_meas_dR0_age=100 % Parameter not set d  dR0_age_mat=[0, 0, 0; 0, 0, 0; 0, 0, 0; 0, 0, 0] % Parameter not set  prm_age_capacity=simscape.enum.tablebattery.prm_age.disabled  OCV_scaling_age_capacity=1.5097e07 % Parameter not set  OCV_offset_age_capacity=8.3625e06 % Parameter not set  temp_exp_age_capacity=0.6011 % Parameter not set V  t_exp_age_capacity=0.75 % Parameter not set  T_age_vec_capacity=[273.15, 298.15, 323.15] % Parameter not set K  dt_age_vec_capacity=[0, 90, 180, 270] % Parameter not set d  dAH_age_vec=[0, 0, 0] % Parameter not set  t_meas_dAH_age=100 % Parameter not set d  dAH_age_mat=[0, 0, 0; 0, 0, 0; 0, 0, 0; 0, 0, 0] % Parameter not set  thermal_port=simscape.enum.thermaleffects.omit  temperature=298.15 % Parameter not set K  thermal_mass=16830 % Parameter assumed J/K  i_specify=off  i_priority=None  i=0 A  i_nominal_specify=off  i_nominal_value=1  i_nominal_unit=A  v_specify=off  v_priority=None  v=0 V  v_nominal_specify=off  v_nominal_value=1  v_nominal_unit=V  stateOfCharge_specify=on  stateOfCharge_priority=High  stateOfCharge=0.5  stateOfCharge_nominal_specify=off  stateOfCharge_nominal_value=1  stateOfCharge_nominal_unit=1  num_cycles_specify=off  num_cycles_priority=High  num_cycles=0  num_cycles_nominal_specify=off  num_cycles_nominal_value=1  num_cycles_nominal_unit=1  cell_temperature_specify=off  cell_temperature_priority=High  cell_temperature=298.15 K  cell_temperature_nominal_specify=off  cell_temperature_nominal_value=1  cell_temperature_nominal_unit=K
      settings: AttributesFormatString=Valence:U27_36XP
  Gain : Gain  Gain=(1/(50*3600))*100
  PS-Simulink Converter : nesl_utility/PS-Simulink Converter  PhysicalDomain=network_engine_domain  SubClassName=ps_output  LeftPortType=input  RightPortType=output  PseudoPeriodic=off  Frequencies=[]  VectorFormat=inherit  Unit=inherit  AffineConversion=off
  Scope : Scope
      settings: ActiveDisplayYMinimum=14.99851  ActiveDisplayYMaximum=15.01344
  To Workspace2 : ToWorkspace  VariableName=SOC  SampleTime=-1
      settings: Save2DSignal=2-D array (concatenate along first dimension)
  Conn2 : PMIOPort  Side=Left
  Conn3 : PMIOPort  Port=2  Side=Right
  tag scope: soc_pct=global
  wires:
  PS-Simulink Converter/1 -> Gain/1
  Gain/1 -> Scope/1, To Workspace2/1, [soc_pct]
  connections:
  Battery/LConn1 -- Conn2/RConn1
  Battery/RConn1 -- Conn3/RConn1
  Battery/LConn2 -- PS-Simulink Converter/LConn1
